simulink model "s6_template"  (R2021b)
settings: Solver=ode4  StartTime=0.0  StopTime=inf  FixedStep=P_sim_dt  RelTol=1e-3
InitFcn:
  | s6_data;
values from neighbouring files (symbols this model uses):
  P_kr = 1/P_ku * sqrt((P_Ti^2*P_omega_d^2 + P_T^2*P_Ti^2*P_omega_d^4) /     (1 + P_Ti^2*P_omega_d^2))    [ex6_1.m]    (also in s6_data.m = 0.3345)
  P_sim_dt = 2e-3    (= 0.002)    [s6_data.m]
  P_T_w = 0.3    [s6_data.m]
  P_Ti = (tan(P_phires_arc - pi + P_Tt*P_omega_d) * P_T * P_omega_d - 1)/     (P_T*P_omega_d^2 + tan(P_phires_arc - pi + P_Tt*P_omega_d) * P_omega_d )    [ex6_1.m]    (also in s6_data.m = 0.2474)
  P_Tt = 0.1    [ex5_1.m]    (also in ex6_1.m; s6_data.m)
  P_u_slow = 0.1    [s6_data.m]
  P_v_fb_border = 0.1    [s6_data.m]
  P_w_breakslen = uint32(length(path.points))    [s6_data.m]
  P_w_periodic = track.periodic    [s6_data.m]
  P_w_points = zeros(SPLINE.Elements(2).Dimensions)    [s6_data.m]
  P_w_ppcoefs = zeros(SPLINE.Elements(3).Dimensions)    [s6_data.m]
  P_w_segments = uint32(zeros(SPLINE.Elements(4).Dimensions))    [s6_data.m]
  points = [p.x + x; s1; s2]    [mbc_clothoid_get_points.m]
  psi = p.psi + ((t.a * t.xe.^2) / 2) - (t.a/2) * (t.xe - x).^2    [mbc_clothoid_get_points.m]
  s1 = p.s1 + integral(fun_cos, 0, xe)    [mbc_clothoid_create.m]
  s2 = p.s2 + integral(fun_sin, 0, xe)    [mbc_clothoid_create.m]
  v_max = 0.5    [s6_data.m]
undefined symbols (not defined in the file or in its folder): breakslen, CarInputsCmdForward, CarInputsCmdHalt, CarInputsCmdReverse, CarInputsCmdSlow, cmd, coefs, P_p_Bf, P_p_Br, P_p_Cf, P_p_Cr, P_p_delta_max, P_p_delta_min, P_p_delta_Tt, P_p_Df, P_p_Dr, P_p_frontaxle_1, P_p_J, P_p_k, P_p_l, P_p_m, P_p_output_Tt, P_p_psi0, P_p_psistd, P_p_rearaxle_1, P_p_s10, P_p_s20, P_p_sstd, P_p_T, P_p_uTt, P_p_v_min, P_p_xvec0, periodic, segments, vmax
libraries: mad_lib_template x1
settings Model: Creator=hmekiedj  LastModifiedBy=exdestruction
settings SolverCC: AlgebraicLoopSolver=TrustRegion
settings DataIOCC: ReturnWorkspaceOutputs=off
settings DebuggingCC: SFMachineParentedDataDiag=warning  ArithmeticOperatorsInVariantConditions=warning
settings SFSimCC: SimUseLocalCustomCode=off  CustomCodeUndefinedFunction=UseInterfaceOnly
settings RTWCC: RTWUseLocalCustomCode=off

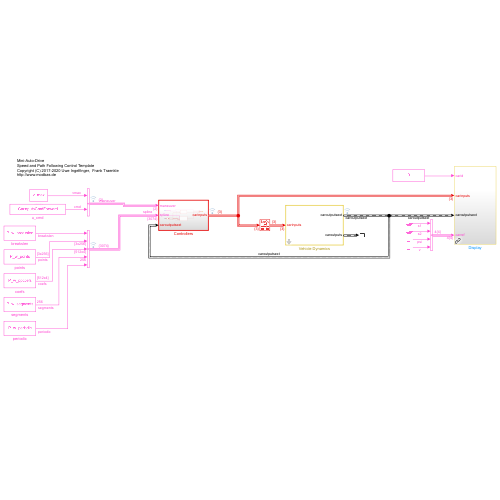
[thumbnail: Simulink's stored preview of the top-level diagram]
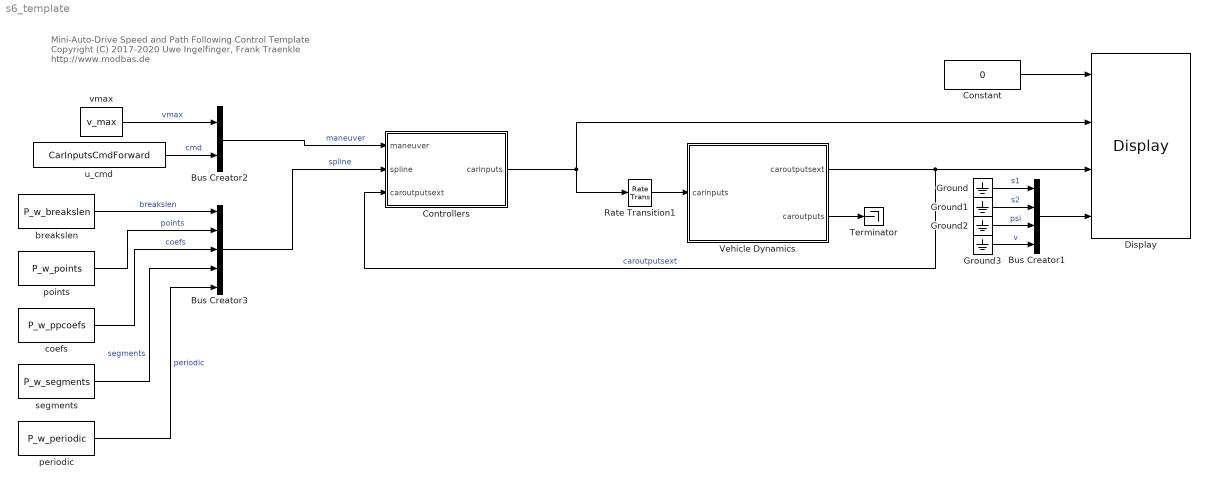
== system s6_template ==
  note: Mini-Auto-Drive
      | Speed and Path Following Control Template
      | Copyright (C) 2017-2020 Uwe Ingelfinger,  Frank Traenkle
      | http://www.modbas.de
  Bus Creator1 : BusCreator  Inputs=4
  Bus Creator2 : BusCreator  Inputs=vmax,cmd
  Bus Creator3 : BusCreator  Inputs=breakslen,points,coefs,segments,periodic  OutDataTypeStr=Bus: SPLINE
  Constant : Constant  Value=0
  Controllers : Subsystem  TreatAsAtomicUnit=on  SystemSampleTime=P_sim_dt
      settings: MinAlgLoopOccurrences=on
  Display : mad_lib_template/Display  SystemSampleTime=-1  VariantActivationTime=update diagram  Latency=0  AutoFrameSizeCalculation=off
  Ground{,1..3} (4 alike) : Ground
  Rate Transition1 : RateTransition  OutPortSampleTime=P_sim_dt
  Terminator : Terminator
  Vehicle Dynamics : Subsystem  TreatAsAtomicUnit=on  mask{P_mask_vec0=P_p_xvec0}
      mask prompts: P_mask_vec0 "Initial vale"
  breakslen : Constant  Value=P_w_breakslen
  coefs : Constant  Value=P_w_ppcoefs
  periodic : Constant  Value=P_w_periodic
  points : Constant  Value=P_w_points
  segments : Constant  Value=P_w_segments
  u_cmd : Constant  Value=CarInputsCmdForward
  vmax : Constant  Value=v_max
  wires:
  Bus Creator1/1 -> Display/4
  Ground/1 -> Bus Creator1/1  "s1"
  Ground1/1 -> Bus Creator1/2  "s2"
  Ground2/1 -> Bus Creator1/3  "psi"
  Ground3/1 -> Bus Creator1/4  "v"
  Vehicle Dynamics/1(caroutputsext) -> Controllers/3(caroutputsext), Display/3  "caroutputsext"
  Rate Transition1/1 -> Vehicle Dynamics/1(carinputs)
  Constant/1 -> Display/1
  Vehicle Dynamics/2(caroutputs) -> Terminator/1
  vmax/1 -> Bus Creator2/1  "vmax"
  u_cmd/1 -> Bus Creator2/2  "cmd"
  Bus Creator2/1 -> Controllers/1(maneuver)  "maneuver"
  Controllers/1(carinputs) -> Rate Transition1/1, Display/2
  Bus Creator3/1 -> Controllers/2(spline)  "spline"
  breakslen/1 -> Bus Creator3/1  "breakslen"
  points/1 -> Bus Creator3/2  "points"
  coefs/1 -> Bus Creator3/3  "coefs"
  segments/1 -> Bus Creator3/4  "segments"
  periodic/1 -> Bus Creator3/5  "periodic"

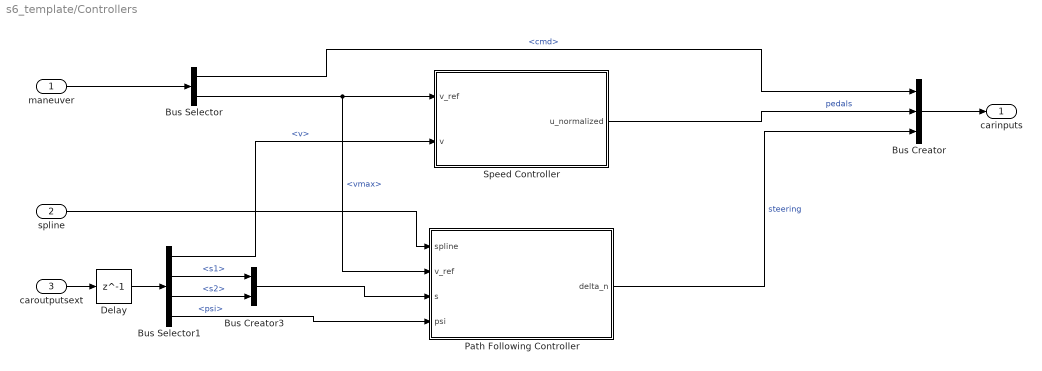
== system s6_template/Controllers ==
  maneuver : Inport
  spline : Inport  Port=2
  caroutputsext : Inport  Port=3
  Bus Creator : BusCreator  Inputs=3
  Bus Creator3 : BusCreator  Inputs=2
  Bus Selector : BusSelector  OutputSignals=cmd,vmax
  Bus Selector1 : BusSelector  OutputSignals=v,s1,s2,psi
  Delay : Delay  DelayLength=1
  Path Following Controller : Subsystem
  Speed Controller : Subsystem
  carinputs : Outport
  wires:
  Bus Selector1/1 -> Speed Controller/2(v)  "<v>"
  Bus Creator3/1 -> Path Following Controller/3(s)
  Bus Selector1/3 -> Bus Creator3/2  "<s2>"
  Bus Selector1/2 -> Bus Creator3/1  "<s1>"
  Bus Selector1/4 -> Path Following Controller/4(psi)  "<psi>"
  Speed Controller/1(u_normalized) -> Bus Creator/2  "pedals"
  caroutputsext/1 -> Delay/1
  maneuver/1 -> Bus Selector/1
  Bus Selector/2 -> Speed Controller/1(v_ref), Path Following Controller/2(v_ref)  "<vmax>"
  Bus Creator/1 -> carinputs/1
  Bus Selector/1 -> Bus Creator/1  "<cmd>"
  Path Following Controller/1(delta_n) -> Bus Creator/3  "steering"
  Delay/1 -> Bus Selector1/1
  spline/1 -> Path Following Controller/1(spline)

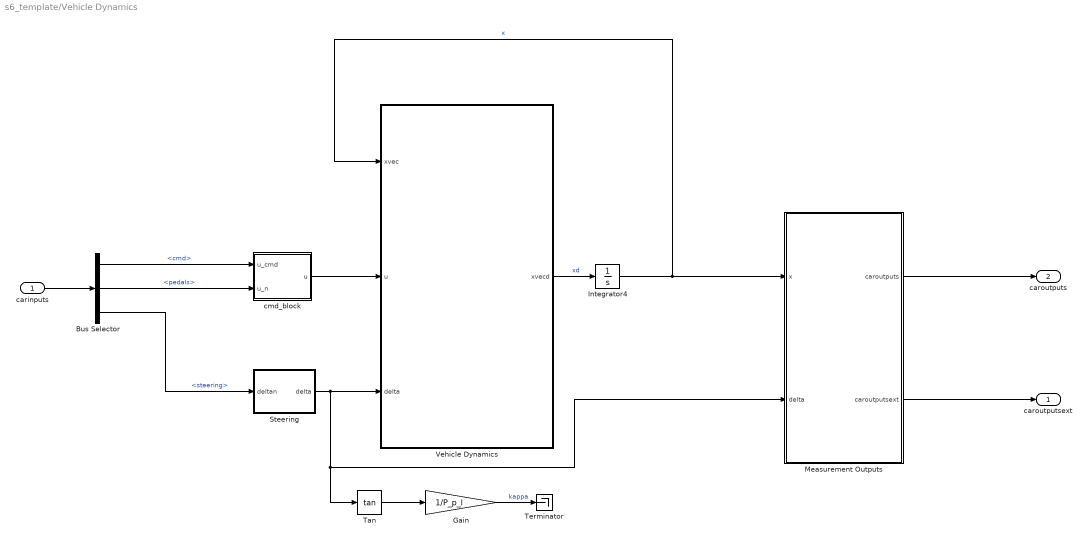
== system s6_template/Vehicle Dynamics ==
  carinputs : Inport
  Bus Selector : BusSelector  OutputSignals=cmd,pedals,steering
  Gain : Gain  Gain=1/P_p_l
  Integrator4 : Integrator  InitialCondition=P_mask_vec0
  Measurement Outputs : Subsystem
  "Steering " : Subsystem
  Tan : Trigonometry  Operator=tan
  Terminator : Terminator
  Vehicle Dynamics : MATLAB Function  TreatAsAtomicUnit=on
  cmd_block : Subsystem
  caroutputsext : Outport  VectorParamsAs1DForOutWhenUnconnected=off
  caroutputs : Outport  Port=2  VectorParamsAs1DForOutWhenUnconnected=off
  wires:
  carinputs/1 -> Bus Selector/1
  cmd_block/1(u) -> Vehicle Dynamics/2(u)
  "Steering "/1(delta) -> Tan/1, Measurement Outputs/2(delta), Vehicle Dynamics/3(delta)
  Vehicle Dynamics/1(xvecd) -> Integrator4/1  "xd"
  Integrator4/1 -> Vehicle Dynamics/1(xvec), Measurement Outputs/1(x)  "x"
  Bus Selector/2 -> cmd_block/2(u_n)  "<pedals>"
  Bus Selector/3 -> "Steering "/1(deltan)  "<steering>"
  Measurement Outputs/1(caroutputs) -> caroutputs/1
  Measurement Outputs/2(caroutputsext) -> caroutputsext/1
  Tan/1 -> Gain/1
  Gain/1 -> Terminator/1  "kappa"
  Bus Selector/1 -> cmd_block/1(u_cmd)  "<cmd>"

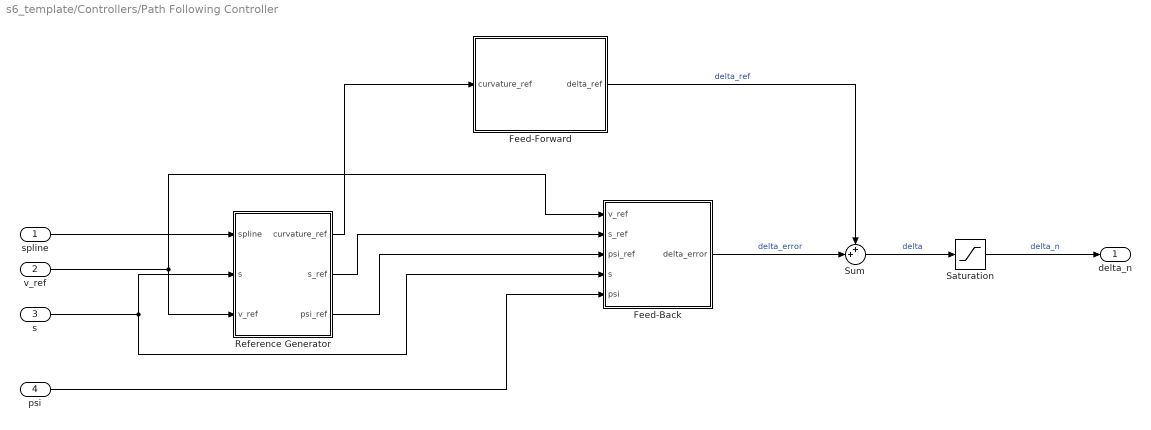
== system s6_template/Controllers/Path Following Controller ==
  spline : Inport
  v_ref : Inport  Port=2
  s : Inport  Port=3
  psi : Inport  Port=4
  Feed-Back : Subsystem
  Feed-Forward : Subsystem
  Reference Generator : Subsystem
  Saturation : Saturate  UpperLimit=1  LowerLimit=-1
  Sum : Sum  Inputs=++|
  delta_n : Outport
  wires:
  Saturation/1 -> delta_n/1  "delta_n"
  Sum/1 -> Saturation/1  "delta"
  Feed-Back/1(delta_error) -> Sum/2  "delta_error"
  Reference Generator/2(s_ref) -> Feed-Back/2(s_ref)
  Reference Generator/3(psi_ref) -> Feed-Back/3(psi_ref)
  s/1 -> Feed-Back/4(s), Reference Generator/2(s)
  psi/1 -> Feed-Back/5(psi)
  Reference Generator/1(curvature_ref) -> Feed-Forward/1(curvature_ref)
  v_ref/1 -> Feed-Back/1(v_ref), Reference Generator/3(v_ref)
  Feed-Forward/1(delta_ref) -> Sum/1  "delta_ref"
  spline/1 -> Reference Generator/1(spline)

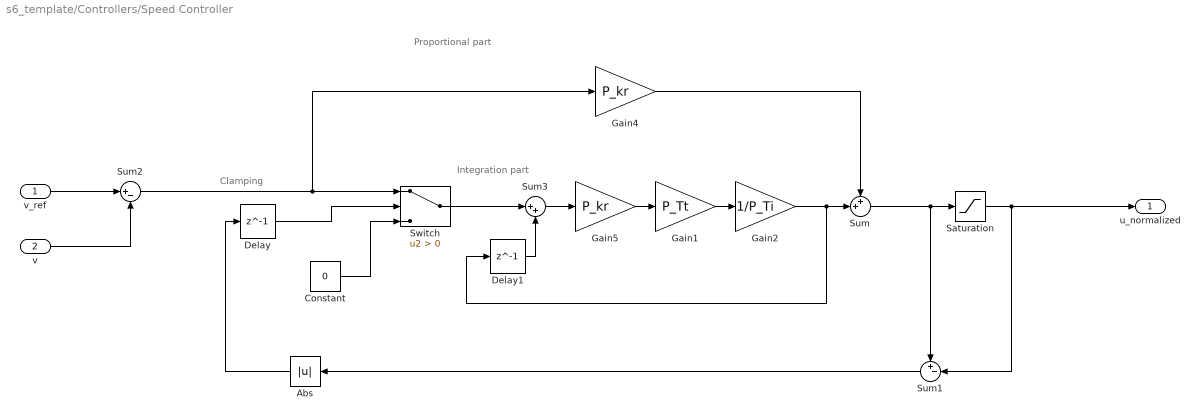
== system s6_template/Controllers/Speed Controller ==
  note: Clamping
  note: Proportional part
  note: Integration part
  v_ref : Inport
  v : Inport  Port=2
  Abs : Abs
  Constant : Constant  Value=0
  Delay : Delay  DelayLength=1  InitialCondition=0
  Delay1 : Delay  DelayLength=1  InitialCondition=0
  Gain1 : Gain  Gain=P_Tt
  Gain2 : Gain  Gain=1/P_Ti
  Gain4 : Gain  Gain=P_kr
  Gain5 : Gain  Gain=P_kr
  Saturation : Saturate  UpperLimit=1  LowerLimit=-1
  Sum : Sum  Inputs=++|
  Sum1 : Sum  Inputs=+-|
  Sum2 : Sum  Inputs=|+-
  Sum3 : Sum  Inputs=|++
  Switch : Switch  Criteria=u2 > Threshold
  u_normalized : Outport
  wires:
  Sum1/1 -> Abs/1
  Sum/1 -> Saturation/1, Sum1/1
  Saturation/1 -> u_normalized/1, Sum1/2
  Sum2/1 -> Gain4/1, Switch/1
  Constant/1 -> Switch/3
  v_ref/1 -> Sum2/1
  v/1 -> Sum2/2
  Delay/1 -> Switch/2
  Abs/1 -> Delay/1
  Gain1/1 -> Gain2/1
  Switch/1 -> Sum3/1
  Delay1/1 -> Sum3/2
  Gain2/1 -> Delay1/1, Sum/2
  Gain4/1 -> Sum/1
  Sum3/1 -> Gain5/1
  Gain5/1 -> Gain1/1

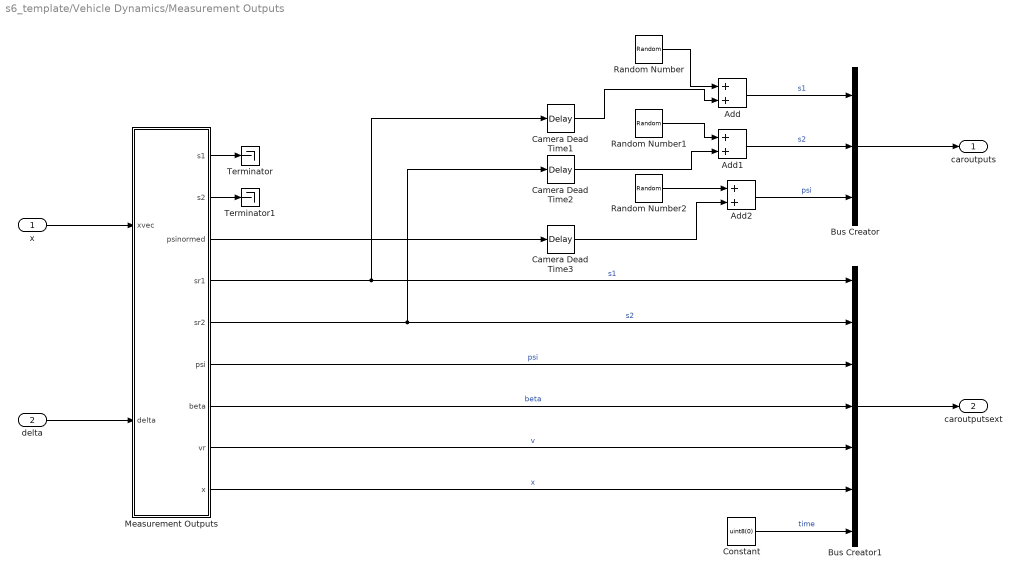
== system s6_template/Vehicle Dynamics/Measurement Outputs ==
  x : Inport
  delta : Inport  Port=2
  Add : Sum
  Add1 : Sum
  Add2 : Sum
  Bus Creator : BusCreator  Inputs=s1,s2,psi  OutDataTypeStr=Bus: CAROUTPUTS  NonVirtualBus=on
  Bus Creator1 : BusCreator  Inputs=7  OutDataTypeStr=Bus: CAROUTPUTSEXT  NonVirtualBus=on
  Camera Dead Time1 : TransportDelay  DelayTime=P_p_output_Tt  InitialOutput=P_p_s10  FixedBuffer=on
  Camera Dead Time2 : TransportDelay  DelayTime=P_p_output_Tt  InitialOutput=P_p_s20  FixedBuffer=on
  Camera Dead Time3 : TransportDelay  DelayTime=P_p_output_Tt  InitialOutput=P_p_psi0  FixedBuffer=on
  Constant : Constant  Value=uint8(0)
  Measurement Outputs : MATLAB Function  TreatAsAtomicUnit=on
  Random Number : RandomNumber  Variance=P_p_sstd^2  SampleTime=P_sim_dt
  Random Number1 : RandomNumber  Variance=P_p_sstd^2  Seed=1  SampleTime=P_sim_dt
  Random Number2 : RandomNumber  Variance=P_p_psistd^2  Seed=2  SampleTime=P_sim_dt
  Terminator : Terminator
  Terminator1 : Terminator
  caroutputs : Outport  VectorParamsAs1DForOutWhenUnconnected=off
  caroutputsext : Outport  Port=2  VectorParamsAs1DForOutWhenUnconnected=off
  wires:
  Measurement Outputs/4(sr1) -> Camera Dead Time1/1, Bus Creator1/1  "s1"
  Measurement Outputs/7(beta) -> Bus Creator1/4  "beta"
  Measurement Outputs/8(vr) -> Bus Creator1/5  "v"
  Measurement Outputs/9(x) -> Bus Creator1/6  "x"
  Measurement Outputs/5(sr2) -> Bus Creator1/2, Camera Dead Time2/1  "s2"
  Bus Creator/1 -> caroutputs/1
  Bus Creator1/1 -> caroutputsext/1
  x/1 -> Measurement Outputs/1(xvec)
  Camera Dead Time1/1 -> Add/2
  Random Number/1 -> Add/1
  Add/1 -> Bus Creator/1  "s1"
  Random Number1/1 -> Add1/1
  Camera Dead Time2/1 -> Add1/2
  Add1/1 -> Bus Creator/2  "s2"
  Camera Dead Time3/1 -> Add2/2
  Random Number2/1 -> Add2/1
  Add2/1 -> Bus Creator/3  "psi"
  delta/1 -> Measurement Outputs/2(delta)
  Measurement Outputs/3(psinormed) -> Camera Dead Time3/1
  Measurement Outputs/6(psi) -> Bus Creator1/3  "psi"
  Constant/1 -> Bus Creator1/7  "time"
  Measurement Outputs/1(s1) -> Terminator/1
  Measurement Outputs/2(s2) -> Terminator1/1

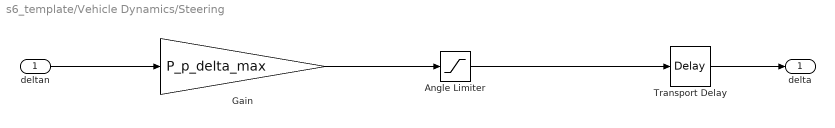
== system s6_template/Vehicle Dynamics/Steering  ==
  deltan : Inport
  Angle Limiter : Saturate  UpperLimit=P_p_delta_max  LowerLimit=P_p_delta_min
  Gain : Gain  Gain=P_p_delta_max
  Transport Delay : TransportDelay  DelayTime=P_p_delta_Tt  FixedBuffer=on
  delta : Outport  VectorParamsAs1DForOutWhenUnconnected=off
  wires:
  deltan/1 -> Gain/1
  Gain/1 -> Angle Limiter/1
  Transport Delay/1 -> delta/1
  Angle Limiter/1 -> Transport Delay/1

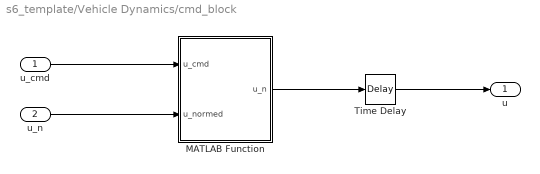
== system s6_template/Vehicle Dynamics/cmd_block ==
  u_cmd : Inport
  u_n : Inport  Port=2
  MATLAB Function : MATLAB Function  TreatAsAtomicUnit=on
  Time Delay : TransportDelay  DelayTime=P_p_uTt  FixedBuffer=on
  u : Outport  VectorParamsAs1DForOutWhenUnconnected=off
  wires:
  Time Delay/1 -> u/1
  MATLAB Function/1(u_n) -> Time Delay/1
  u_n/1 -> MATLAB Function/2(u_normed)
  u_cmd/1 -> MATLAB Function/1(u_cmd)

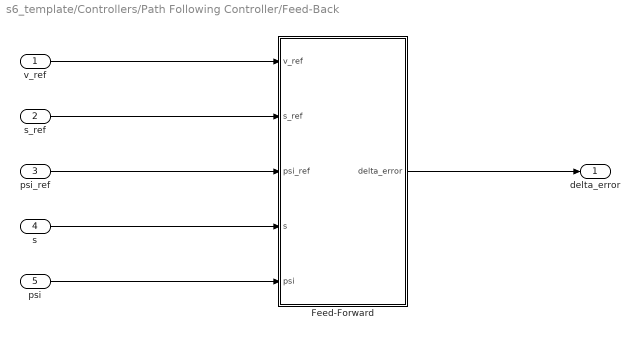
== system s6_template/Controllers/Path Following Controller/Feed-Back ==
  v_ref : Inport
  s_ref : Inport  Port=2
  psi_ref : Inport  Port=3
  s : Inport  Port=4
  psi : Inport  Port=5
  Feed-Forward : MATLAB Function  TreatAsAtomicUnit=on
  delta_error : Outport
  wires:
  Feed-Forward/1(delta_error) -> delta_error/1
  v_ref/1 -> Feed-Forward/1(v_ref)
  s_ref/1 -> Feed-Forward/2(s_ref)
  psi_ref/1 -> Feed-Forward/3(psi_ref)
  s/1 -> Feed-Forward/4(s)
  psi/1 -> Feed-Forward/5(psi)

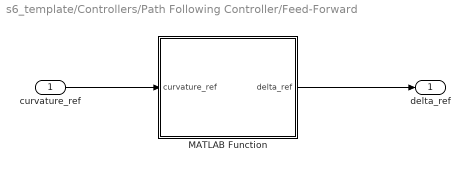
== system s6_template/Controllers/Path Following Controller/Feed-Forward ==
  curvature_ref : Inport
  MATLAB Function : MATLAB Function  TreatAsAtomicUnit=on
  delta_ref : Outport
  wires:
  curvature_ref/1 -> MATLAB Function/1(curvature_ref)
  MATLAB Function/1(delta_ref) -> delta_ref/1

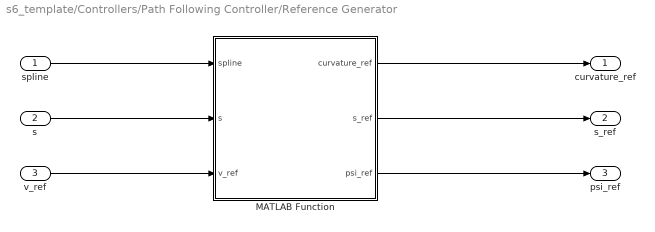
== system s6_template/Controllers/Path Following Controller/Reference Generator ==
  spline : Inport
  s : Inport  Port=2
  v_ref : Inport  Port=3
  MATLAB Function : MATLAB Function  TreatAsAtomicUnit=on
  curvature_ref : Outport
  s_ref : Outport  Port=2
  psi_ref : Outport  Port=3
  wires:
  v_ref/1 -> MATLAB Function/3(v_ref)
  s/1 -> MATLAB Function/2(s)
  MATLAB Function/1(curvature_ref) -> curvature_ref/1
  MATLAB Function/2(s_ref) -> s_ref/1
  MATLAB Function/3(psi_ref) -> psi_ref/1
  spline/1 -> MATLAB Function/1(spline)

== matlab function s6_template/Controllers/Path Following Controller/Feed-Back/Feed-Forward ==
  data: v_ref input; delta_error output; s_ref input; psi_ref input; s input; psi input; P_v_fb_border parameter; P_p_l parameter; P_T_w parameter
function delta_error = feed_back(v_ref, s_ref, psi_ref, s, psi, P_v_fb_border, P_p_l, P_T_w)


if abs(v_ref) < P_v_fb_border
    v_ref = sign(v_ref) .* P_v_fb_border;
end

normal_vector_ref = [-sin(psi_ref); cos(psi_ref)];
psi_error = psi - psi_ref;
psi_error = mod(psi_error, 2*pi);
if psi_error > pi
    psi_error = psi_error - 2*pi;
end
s_c2e = (s - s_ref)' * normal_vector_ref;
delta_error = -(P_p_l*s_c2e)/(P_T_w * v_ref)^2 - (2*P_p_l*psi_error)/(P_T_w*v_ref);

% delta_error = mod(delta_error, pi);

== matlab function s6_template/Controllers/Path Following Controller/Feed-Forward/MATLAB Function ==
  data: delta_ref output; curvature_ref input; P_p_l parameter
function delta_ref = feed_forward(curvature_ref, P_p_l)

delta_ref = atan(P_p_l * curvature_ref);

== matlab function s6_template/Controllers/Path Following Controller/Reference Generator/MATLAB Function ==
  data: spline input; s input; v_ref input; curvature_ref output; s_ref output; psi_ref output; P_Tt parameter
function [curvature_ref, s_ref, psi_ref] = reference_generator(spline, s, v_ref, P_Tt)


[w, ~]  = mbc_spline_get_reference(s, spline.breakslen, spline.points, spline.coefs, spline.periodic, v_ref, P_Tt);

s_ref = [w(3); w(4)];
psi_ref = w(2);
curvature_ref = w(5);

== matlab function s6_template/Vehicle Dynamics/Measurement Outputs/Measurement Outputs ==
  data: xvec input; delta input; s1 output; s2 output; psinormed output; sr1 output; sr2 output; psi output; beta output; vr output; x output; P_p_rearaxle_1 parameter; P_p_v_min parameter; P_p_l parameter
function [s1, s2, psinormed, sr1, sr2, psi, beta, vr, x] = outputs(xvec, delta, P_p_rearaxle_1, P_p_v_min, P_p_l)
%#codegen
vc1 = xvec(1);
s1 = xvec(2);
s2 = xvec(3);
psi = xvec(4);
x = xvec(7);

psinormed = mod(psi, 2*pi);
if psinormed > pi
    psinormed = psinormed - 2*pi;
end
beta = 0;
sr1 = s1 - P_p_rearaxle_1 * cos(psi);
sr2 = s2 - P_p_rearaxle_1 * sin(psi);
vr = vc1;
end

== matlab function s6_template/Vehicle Dynamics/Vehicle Dynamics ==
  data: xvec input; u input; xvecd output; delta input; P_p_Br parameter; P_p_Bf parameter; P_p_Cr parameter; P_p_Cf parameter; P_p_Dr parameter; P_p_Df parameter; P_p_rearaxle_1 parameter; P_p_frontaxle_1 parameter; P_p_m parameter; P_p_J parameter; P_p_k parameter; P_p_T parameter; P_p_v_min parameter; P_p_l parameter
function xvecd = dynamics(xvec, u, delta, P_p_Br, P_p_Bf, P_p_Cr, P_p_Cf, P_p_Dr, P_p_Df, ...
    P_p_rearaxle_1, P_p_frontaxle_1, P_p_m, P_p_J, P_p_k, P_p_T, P_p_v_min, P_p_l)
%#codegen

vc1 = xvec(1);
psi = xvec(4);
psid = xvec(5);
vc2 = xvec(6);

if abs(vc1) > P_p_v_min % avoid model singularity at zero speed
    %% bicycle model with Magic Tire
    spsi = sin(psi);
    cpsi = cos(psi);
    sdelta = sin(delta);
    cdelta = cos(delta);
    
    % wheel slip angles
    alphaf = -atan2(vc2 + P_p_frontaxle_1 * psid, vc1) + delta;
    alphar = -atan2(vc2 - P_p_rearaxle_1 * psid, vc1);
    % wheel forces
    Ff = P_p_Df * sin(P_p_Cf * atan(P_p_Bf * alphaf));
    Fr = P_p_Dr * sin(P_p_Cr * atan(P_p_Br * alphar));    
    % logitudinal dynamics (momentum balance)
    vc1d = (-Ff * sdelta + P_p_m * vc2 * psid) / P_p_m ...
            - vc1/P_p_T + P_p_k/P_p_T * u;
    % kinematics
    s1d = vc1 * cpsi - vc2 * spsi;
    s2d = vc1 * spsi + vc2 * cpsi;
    % rotational dynamics (moment of momentum balance)
    psidd = (Ff * P_p_frontaxle_1 * cdelta - Fr * P_p_rearaxle_1) / P_p_J;
    % lateral dynamics (momentum balance)
    vc2d = (Ff * cdelta + Fr - P_p_m * vc1 * psid)/P_p_m;
    % driven arc length of rear axle center
    xd = vc1;
else % near zero speed
    %% longitudinal dynamics of rear axle
    a = P_p_rearaxle_1;
    l = P_p_l;
    spsi = sin(psi);
    cpsi = cos(psi);
    tdelta = tan(delta);
    vc2 = a/l * vc1 * tdelta;
    vc1d = (-vc1 + P_p_k * u) / P_p_T; % -(a^2+P_p_J/P_p-m)/l^2*vc1*tdelta*deltad
    s1d = vc1 * cpsi - vc2 * spsi;
    s2d = vc1 * spsi + vc2 * cpsi;
    psid = vc1 / l * tdelta;
    psidd = 0; % vc1d / l * tdelta + vc1/l * deltad * (1 + tdelta*delta)
    vc2d = 0 ; % a * psidd;
    xd = vc1;
end
    
xvecd = [ vc1d; s1d; s2d; psid; psidd; vc2d; xd ];
end

== matlab function s6_template/Vehicle Dynamics/cmd_block/MATLAB Function ==
  data: u_cmd input; u_n output; u_normed input; P_u_slow parameter; CarInputsCmdSlow parameter; CarInputsCmdReverse parameter; CarInputsCmdForward parameter; CarInputsCmdHalt parameter
function u_n = fcn(u_cmd, u_normed, P_u_slow, CarInputsCmdSlow,  CarInputsCmdReverse, CarInputsCmdForward, CarInputsCmdHalt)

u_n = u_normed;
if u_cmd == CarInputsCmdHalt
    u_n = 0;
elseif u_cmd == CarInputsCmdForward
    if u_normed > 1
        u_n = 1;
    elseif u_normed < 0
        u_n = 0;
    end
elseif u_cmd == CarInputsCmdReverse
    if u_normed > 0
        u_n = 0;
    elseif u_normed < -1
        u_n = -1;
    end
elseif u_cmd == CarInputsCmdSlow
    u_n = P_u_slow * sign(u_normed);
end
